simulink model "Projekt_ABS_Sim_4_3"  (R2024b)
settings: Solver=VariableStepAuto  StartTime=0.0  StopTime=20  RelTol=1e-3
values from neighbouring files (symbols this model uses):
  c1 = 0.857    [Projekt_ABS.m]
  c11 = 1.2801    [Projekt_ABS.m]
  c2 = 33.822    [Projekt_ABS.m]
  c22 = 23.99    [Projekt_ABS.m]
  c3 = 0.347    [Projekt_ABS.m]
  c33 = 0.52    [Projekt_ABS.m]
  c4 = 0.035    [Projekt_ABS.m]
  c44 = 0.03    [Projekt_ABS.m]
  g = 9.81    [Projekt_ABS.m]
  J = 1.6    [Projekt_ABS.m]
  m = 1200    [Projekt_ABS.m]
  Mb = 900    [Projekt_ABS.m]
  R = 0.315    [Projekt_ABS.m]
  V0 = 40    [Projekt_ABS.m]
undefined symbols (not defined in the file or in its folder): DiscIntNeverNeededParam
libraries: simulink x2
settings Model: Creator=abc  LastModifiedBy=abc

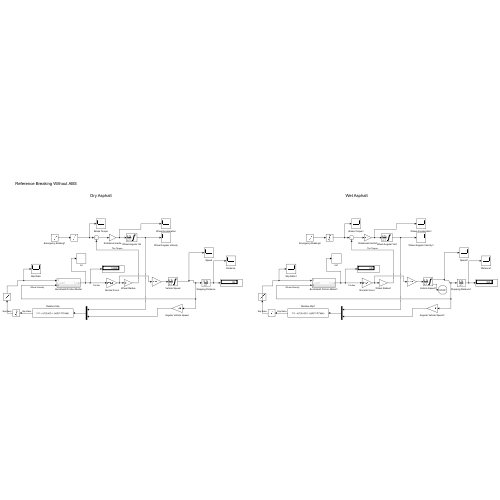
[thumbnail: Simulink's stored preview of the top-level diagram]
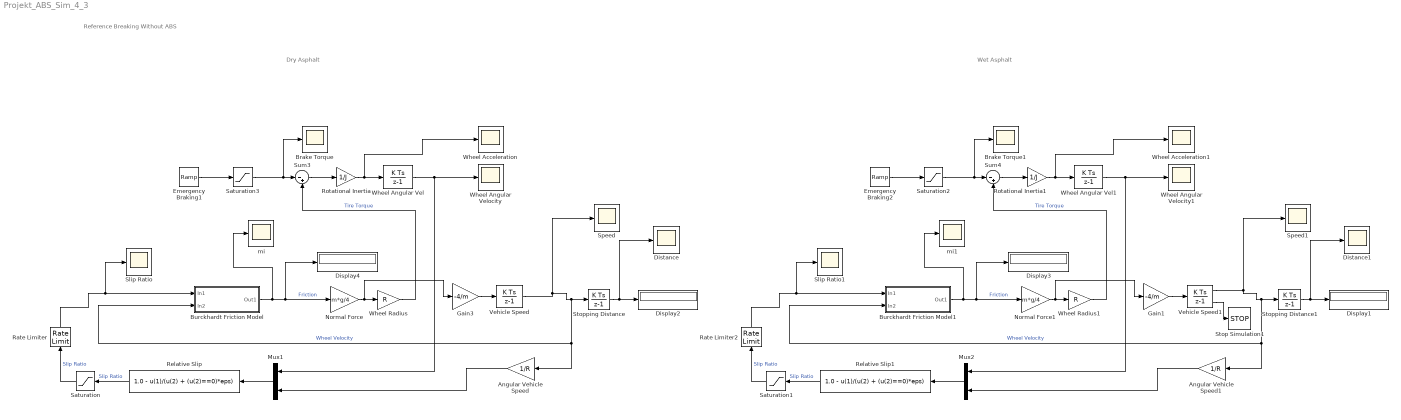
== system Projekt_ABS_Sim_4_3 ==
  note: Dry Asphalt
  note: Reference Breaking Without ABS
  note: Wet Asphalt
  Angular Vehicle Speed : Gain  Gain=1/R
  Angular Vehicle Speed1 : Gain  Gain=1/R
  Brake Torque : Scope
  Brake Torque1 : Scope
  Burckhardt Friction Model : Subsystem
  Burckhardt Friction Model1 : Subsystem
  Display{1..4} (4 alike) : Display
  Distance : Scope
  Distance1 : Scope
  Emergency Braking1 : simulink/Sources/Ramp  slope=Mb*2  start=0  InitialOutput=0
  Emergency Braking2 : simulink/Sources/Ramp  slope=Mb*2  start=0  InitialOutput=0
  Gain1 : Gain  Gain=-4/m
  Gain3 : Gain  Gain=-4/m
  Mux1 : Mux  Inputs=2
  Mux2 : Mux  Inputs=2
  Normal Force : Gain  Gain=m*g/4
  Normal Force1 : Gain  Gain=m*g/4
  Rate Limiter : RateLimiter  RisingSlewLimit=1.5  FallingSlewLimit=-1.5  SampleTimeMode=inherited
  Rate Limiter2 : RateLimiter  RisingSlewLimit=1.5  FallingSlewLimit=-1.5  SampleTimeMode=inherited
  Relative Slip : Fcn  Expr=1.0 - u(1)/(u(2) + (u(2)==0)*eps)
  Relative Slip1 : Fcn  Expr=1.0 - u(1)/(u(2) + (u(2)==0)*eps)
  Rotational Inertia : Gain  Gain=1/J
  Rotational Inertia1 : Gain  Gain=1/J
  Saturation : Saturate  UpperLimit=1  LowerLimit=0
  Saturation1 : Saturate  UpperLimit=1  LowerLimit=0
  Saturation2 : Saturate  UpperLimit=Mb  LowerLimit=0
  Saturation3 : Saturate  UpperLimit=Mb  LowerLimit=0
  Slip Ratio : Scope
  Slip Ratio1 : Scope
  Speed : Scope
  Speed1 : Scope
  Stop Simulation1 : Stop
  Stopping Distance : DiscreteIntegrator  SampleTime=0.01  ICPrevOutput=DiscIntNeverNeededParam  ICPrevScaledInput=DiscIntNeverNeededParam
  Stopping Distance1 : DiscreteIntegrator  SampleTime=0.01  ICPrevOutput=DiscIntNeverNeededParam  ICPrevScaledInput=DiscIntNeverNeededParam
  Sum3 : Sum  Inputs=|-+
  Sum4 : Sum  Inputs=|-+
  Vehicle Speed : DiscreteIntegrator  InitialCondition=V0  SampleTime=0.01  LimitOutput=on  UpperSaturationLimit=1000  LowerSaturationLimit=0  ICPrevOutput=DiscIntNeverNeededParam  ICPrevScaledInput=DiscIntNeverNeededParam
  Vehicle Speed1 : DiscreteIntegrator  InitialCondition=V0  SampleTime=0.01  LimitOutput=on  UpperSaturationLimit=1000  LowerSaturationLimit=0  ShowSaturationPort=on  ICPrevOutput=DiscIntNeverNeededParam  ICPrevScaledInput=DiscIntNeverNeededParam
  Wheel Acceleration : Scope
  Wheel Acceleration1 : Scope
  Wheel Angular Vel : DiscreteIntegrator  InitialCondition=V0/R  SampleTime=0.01  LimitOutput=on  UpperSaturationLimit=1000  LowerSaturationLimit=0  ICPrevOutput=DiscIntNeverNeededParam  ICPrevScaledInput=DiscIntNeverNeededParam
  Wheel Angular Vel1 : DiscreteIntegrator  InitialCondition=V0/R  SampleTime=0.01  LimitOutput=on  UpperSaturationLimit=1000  LowerSaturationLimit=0  ICPrevOutput=DiscIntNeverNeededParam  ICPrevScaledInput=DiscIntNeverNeededParam
  Wheel Angular Velocity : Scope
  Wheel Angular Velocity1 : Scope
  Wheel Radius : Gain  Gain=R
  Wheel Radius1 : Gain  Gain=R
  mi : Scope
  mi1 : Scope
  wires:
  Sum3/1 -> Rotational Inertia/1
  Vehicle Speed/1 -> Speed/1, Stopping Distance/1, Burckhardt Friction Model/2(In2), Angular Vehicle Speed/1  "Wheel Velocity"
  Stopping Distance/1 -> Distance/1, Display2/1
  Wheel Angular Vel/1 -> Wheel Angular Velocity/1, Mux1/1
  Relative Slip/1 -> Saturation/1  "Slip Ratio"
  Burckhardt Friction Model/1(Out1) -> mi/1, Display4/1, Normal Force/1  "Friction"
  Mux1/1 -> Relative Slip/1
  Normal Force/1 -> Gain3/1, Wheel Radius/1
  Rotational Inertia/1 -> Wheel Angular Vel/1, Wheel Acceleration/1
  Wheel Radius/1 -> Sum3/2  "Tire Torque"
  Angular Vehicle Speed/1 -> Mux1/2
  Saturation3/1 -> Brake Torque/1, Sum3/1
  Gain3/1 -> Vehicle Speed/1
  Rate Limiter/1 -> Slip Ratio/1, Burckhardt Friction Model/1(In1)
  Saturation/1 -> Rate Limiter/1  "Slip Ratio"
  Emergency Braking1/1 -> Saturation3/1
  Vehicle Speed1/2 -> Stop Simulation1/1
  Sum4/1 -> Rotational Inertia1/1
  Burckhardt Friction Model1/1(Out1) -> mi1/1, Display3/1, Normal Force1/1  "Friction"
  Saturation1/1 -> Rate Limiter2/1  "Slip Ratio"
  Vehicle Speed1/1 -> Stopping Distance1/1, Burckhardt Friction Model1/2(In2), Angular Vehicle Speed1/1, Speed1/1  "Wheel Velocity"
  Angular Vehicle Speed1/1 -> Mux2/2
  Saturation2/1 -> Brake Torque1/1, Sum4/1
  Wheel Radius1/1 -> Sum4/2  "Tire Torque"
  Gain1/1 -> Vehicle Speed1/1
  Rotational Inertia1/1 -> Wheel Angular Vel1/1, Wheel Acceleration1/1
  Rate Limiter2/1 -> Slip Ratio1/1, Burckhardt Friction Model1/1(In1)
  Emergency Braking2/1 -> Saturation2/1
  Normal Force1/1 -> Gain1/1, Wheel Radius1/1
  Stopping Distance1/1 -> Distance1/1, Display1/1
  Mux2/1 -> Relative Slip1/1
  Wheel Angular Vel1/1 -> Wheel Angular Velocity1/1, Mux2/1
  Relative Slip1/1 -> Saturation1/1  "Slip Ratio"

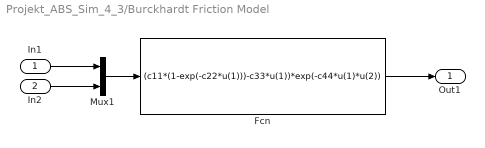
== system Projekt_ABS_Sim_4_3/Burckhardt Friction Model ==
  In1 : Inport
  In2 : Inport  Port=2
  Fcn : Fcn  Expr=(c11*(1-exp(-c22*u(1)))-c33*u(1))*exp(-c44*u(1)*u(2))
  Mux1 : Mux  Inputs=2
  Out1 : Outport
  wires:
  In2/1 -> Mux1/2
  Mux1/1 -> Fcn/1
  In1/1 -> Mux1/1
  Fcn/1 -> Out1/1

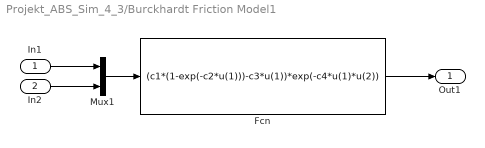
== system Projekt_ABS_Sim_4_3/Burckhardt Friction Model1 ==
  In1 : Inport
  In2 : Inport  Port=2
  Fcn : Fcn  Expr=(c1*(1-exp(-c2*u(1)))-c3*u(1))*exp(-c4*u(1)*u(2))
  Mux1 : Mux  Inputs=2
  Out1 : Outport
  wires:
  In2/1 -> Mux1/2
  Mux1/1 -> Fcn/1
  In1/1 -> Mux1/1
  Fcn/1 -> Out1/1
